simulink model "scarsModel"  (R2019b)
settings: Solver=ode14x  StartTime=0.0  StopTime=2000  FixedStep=0.1  MaxStep=1  MinStep=dT  RelTol=1e-3
model workspace (MAT data in the model file):
  actuators = 0
undefined symbols (not defined in the file): decsec, decstart, forcesBody, gyro, initMoments, L_mt, mag_sat, momentsBody, mt_gain, R_mt, refEuler, refVel, sun_position, TFinal, thruster, WMM2000
libraries: scars_library x15, simulink x3, vrlib x3, simulink_extras x2, aerolibnav x2, aerolibgravity2 x2, sharedtransform x2, aerolibutil x2, sharedutil x2
settings Model: OrderedModelArguments=off  Creator=asmialek  LastModifiedBy=asmialek
settings DataIOCC: SaveFormat=Array  ReturnWorkspaceOutputsName=scars_out

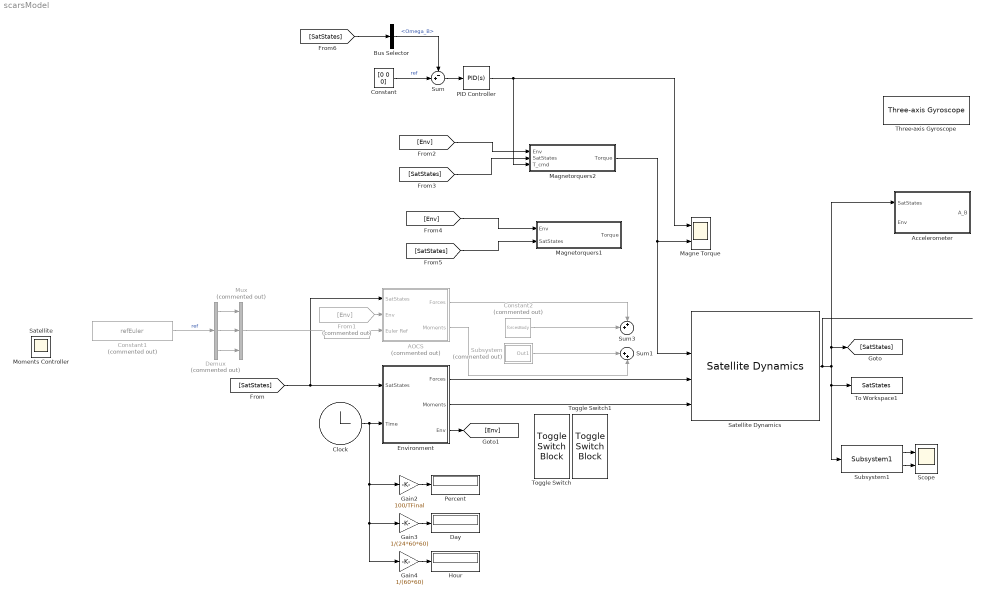
== system scarsModel ==
  AOCS : Subsystem  Commented=on
  Accelerometer : Subsystem
  Bus Selector : BusSelector  OutputSignals=Omega_B
  Clock : Clock
  Constant : Constant  Value=[0 0 0]
  Constant1 : Constant  Commented=on  Value=refEuler
  Constant2 : Constant  Commented=on  Value=forcesBody
  Day : Display
  Demux : Demux  Commented=on  Outputs=3
  "Environment " : Subsystem
  From1 : From  Commented=on  GotoTag=Env
  Gain2 : Gain  Gain=100/TFinal
  Gain3 : Gain  Gain=1/(24*60*60)
  Gain4 : Gain  Gain=1/(60*60)
  Hour : Display
  Magne Torque : Scope  NumInputPorts=2
  Magnetorquers1 : Subsystem
  Magnetorquers2 : Subsystem
  Mux : Mux  Commented=on  Inputs=3
  PID Controller : simulink/Continuous/PID Controller  Controller=PID  Form=Parallel  TimeDomain=Continuous-time  SampleTime=-1  IntegratorMethod=Forward Euler  FilterMethod=Forward Euler  ControllerParametersSource=internal  P=0.01  I=0  D=0.1  UseFilter=on  N=100  TunerSelectOption=Transfer Function Based (PID Tuner App)  InitialConditionSource=internal  InitialConditionForIntegrator=0  InitialConditionForFilter=0  DifferentiatorICPrevScaledInput=0  ExternalReset=none  TrackingMode=off  Kt=1  LimitOutput=off  UpperSaturationLimit=inf  LowerSaturationLimit=-inf  LinearizeAsGain=on  AntiWindupMode=none  Kb=1  POutMin=[]  POutMax=[]  IOutMin=[]  IOutMax=[]  DOutMin=[]  DOutMax=[]  NOutMin=[]  NOutMax=[]  SumOutMin=[]  SumOutMax=[]  SaturationOutMin=[]  SaturationOutMax=[]  PParamMin=[]  PParamMax=[]  IParamMin=[]  IParamMax=[]  DParamMin=[]  DParamMax=[]  NParamMin=[]  NParamMax=[]  KbParamMin=[]  KbParamMax=[]  KtParamMin=[]  KtParamMax=[]  KbOutMin=[]  KbOutMax=[]  KtOutMin=[]  KtOutMax=[]  IntegratorOutMin=[]  IntegratorOutMax=[]  FilterOutMin=[]  FilterOutMax=[]  SumI1OutMin=[]  SumI1OutMax=[]  SumI2OutMin=[]  SumI2OutMax=[]  SumI3OutMin=[]  SumI3OutMax=[]  SumI4OutMin=[]  SumI4OutMax=[]  SumDOutMin=[]  SumDOutMax=[]  DifferentiatorOutMin=[]  DifferentiatorOutMax=[]  FilterDiffOutCoefMin=[]  FilterDiffOutCoefMax=[]  ReciprocalOutMin=[]  ReciprocalOutMax=[]  SumDenOutMin=[]  SumDenOutMax=[]  SumNumOutMin=[]  SumNumOutMax=[]  DivideOutMin=[]  DivideOutMax=[]  IntegratorContinuousStateAttributes=''  IntegratorStateMustResolveToSignalObject=off  IntegratorRTWStateStorageClass=Auto  FilterContinuousStateAttributes=''  FilterStateMustResolveToSignalObject=off  FilterRTWStateStorageClass=Auto  ParallelPVariant=InternalParameters  IdealPVariant=Disabled  IVariant=InternalParameters  DVariant=InternalParameters  IntegratorVariant=Continuous  SatVariant=Disabled  AWVariant=Passthrough  PCopyVariant=Disabled  TRVariant=Disabled  FdbkBlocksVariant=Forward  IdealPFdbkVariant=Disabled  SatFdbkVariant=Disabled  DerivativeFilterVariant=ContFilter  NVariant=InternalParameters  NCopyVariant=Disabled  FilterICVariant=InternalICsFilter  IntegratorICVariant=InternalICs  ExternalResetVariant=Disabled  TRSumVariant=Passthrough  SumFdbkVariant=Disabled  SumVariant=Sum_PID
  Percent : Display
  Satellite Dynamics : scars_library/Advanced/Satellite Dynamics  Parameter4=Keplerian Elements  epoch=0  mass=0  a=6356e3+400e3  e=0  incl=0  RA=0  w=0  TA=0  initEuler=[0 0 0]  initEulerRates=[0 0 0]  TA_copy=0  TA_copy_copy=0  TA_copy_copy_copy=[10 25]  TA_copy_copy_copy_copy=[10 25]  initEuler_copy=[0 0 0]  initEulerRates_copy=[0 0 0]
      link override Moments Switch/Moments: Value=1
  Scope : Scope  NumInputPorts=2
  Subsystem : Subsystem  Commented=on
  Subsystem1 : scars_library/Subsystem1  SystemSampleTime=-1  Latency=0  AutoFrameSizeCalculation=off
  Sum : Sum  Inputs=-+|
  Sum1 : Sum  Inputs=|++
  Sum3 : Sum  Inputs=++|
  Three-axis Gyroscope : aerolibnav/Three-axis Gyroscope  dtype_g=on  w_g=190  z_g=0.707  g_sf_cc=[1 0 0; 0 1 0; 0 0 1]  g_bias=[0 0 0]  g_sen=[0 0 0]  g_Ts=0  g_rand=on  g_seeds=[23093 23094 23095]  g_pow=[0.0001 0.0001 0.0001]  g_sat="[-inf  -inf  -inf  inf inf inf]"
      settings: SourceProductName=Aerospace Blockset  SourceProductBaseCode=AE
  To Workspace1 : ToWorkspace  VariableName=SatStates  SaveFormat=Timeseries  SampleTime=-1
  Toggle Switch : ToggleSwitchBlock
      settings: Values={{'Off', 'On'}, [0 1]}
  Toggle Switch1 : ToggleSwitchBlock
      settings: Values={{'Off', 'On'}, [0 1]}
  Moments Controller : Scope
  Satellite : Scope
  wires:
  Constant2/1 -> Sum3/2
  [SatStates] -> AOCS/1(SatStates), "Environment "/1(SatStates)
  "Environment "/1(Forces) -> Satellite Dynamics/3
  "Environment "/2(Moments) -> Satellite Dynamics/4
  Subsystem/1(Out1) -> Sum1/1
  Clock/1 -> Gain4/1, Gain3/1, Gain2/1, "Environment "/2(Time)
  "Environment "/3(Env) -> [Env]
  From1/1 -> AOCS/2(Env)
  AOCS/1(Forces) -> Sum3/1
  AOCS/2(Moments) -> Sum1/2
  Gain2/1 -> Percent/1
  Gain3/1 -> Day/1
  Gain4/1 -> Hour/1
  Constant1/1 -> Demux/1  "ref"
  Demux/2 -> Mux/2
  Demux/3 -> Mux/3
  Demux/1 -> Mux/1
  Mux/1 -> AOCS/3(Euler Ref)
  [Env] -> Magnetorquers1/1(Env)
  [SatStates] -> Magnetorquers1/2(SatStates)
  [SatStates] -> Magnetorquers2/2(SatStates)
  [Env] -> Magnetorquers2/1(Env)
  Constant/1 -> Sum/2  "ref"
  Sum/1 -> PID Controller/1
  Bus Selector/1 -> Sum/1  "<Omega_B>"
  [SatStates] -> Bus Selector/1
  Magnetorquers2/1(Torque) -> Satellite Dynamics/2, Magne Torque/2
  PID Controller/1 -> Magne Torque/1, Magnetorquers2/3(T_cmd)
  Subsystem1/2 -> Scope/2
  Subsystem1/1 -> Scope/1
  Satellite Dynamics/1 -> Subsystem1/1, To Workspace1/1, Accelerometer/1(SatStates), [SatStates]

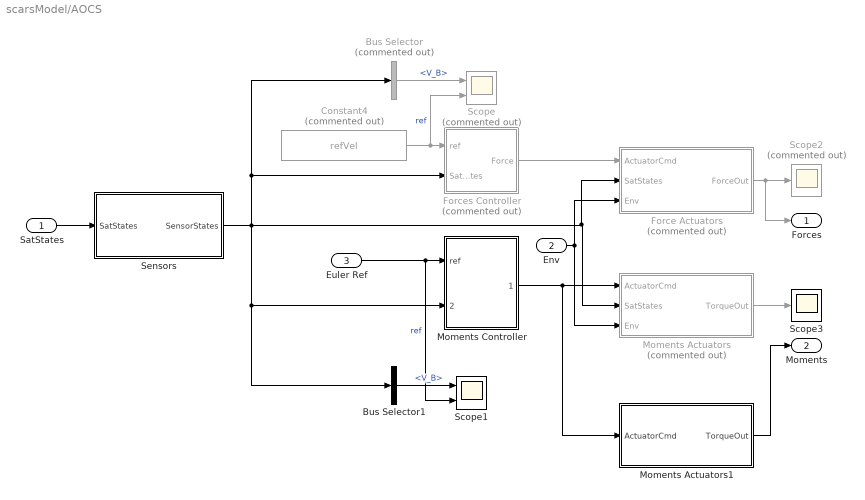
== system scarsModel/AOCS ==
  SatStates : Inport
  Env : Inport  Port=2
  Euler Ref : Inport  Port=3
  Bus Selector : BusSelector  Commented=on  OutputSignals=V_B
  Bus Selector1 : BusSelector  OutputSignals=V_B
  Constant4 : Constant  Commented=on  Value=refVel
  Force Actuators : Subsystem  Commented=on
  Forces Controller : Subsystem  Commented=on
  Moments Actuators : Subsystem  Commented=on
  Moments Actuators1 : Subsystem
  Moments Controller : Subsystem
  Scope : Scope  Commented=on  NumInputPorts=2
  Scope1 : Scope  NumInputPorts=2
  Scope2 : Scope  Commented=on
  Scope3 : Scope
  Sensors : Subsystem
  Forces : Outport
  Moments : Outport  Port=2
  wires:
  Force Actuators/1(ForceOut) -> Forces/1, Scope2/1
  SatStates/1 -> Sensors/1(SatStates)
  Constant4/1 -> Scope/2, Forces Controller/1(ref)  "ref"
  Forces Controller/1(Force) -> Force Actuators/1(ActuatorCmd)
  Euler Ref/1 -> Scope1/2, Moments Controller/1(ref)  "ref"
  Bus Selector/1 -> Scope/1  "<V_B>"
  Bus Selector1/1 -> Scope1/1  "<V_B>"
  Moments Actuators/1(TorqueOut) -> Scope3/1
  Sensors/1(SensorStates) -> Bus Selector/1, Forces Controller/2(SatStates), Force Actuators/2(SatStates), Moments Actuators/2(SatStates), Bus Selector1/1, Moments Controller/2(SatStates)
  Env/1 -> Force Actuators/3(Env), Moments Actuators/3(Env)
  Moments Controller/1(Torque) -> Moments Actuators1/1(ActuatorCmd), Moments Actuators/1(ActuatorCmd)
  Moments Actuators1/1(TorqueOut) -> Moments/1

== system scarsModel/Accelerometer ==
  SatStates : Inport
  Bus Element In : Inport  Port=2  PortName=Env  Element=Gravitational Force [N]
  Bus Selector : BusSelector  OutputSignals=A_B,Omega_B,dOmega_B/dt
  Constant : Constant  Value=[0 0 0]
  Three-axis Accelerometer : aerolibnav/Three-axis Accelerometer  units=Metric (MKS)  acc=[0 0 0]  gtype=on  dtype_a=on  w_a=190  z_a=0.707  a_sf_cc=[1 0 0; 0 1 0; 0 0 1]  a_bias=[0 0 0]  a_Ts=0  a_rand=on  a_seeds=[23093 23094 23095]  a_pow=[0.001 0.001 0.001]  a_sat="[-inf  -inf  -inf  inf inf inf]"
      settings: SourceProductName=Aerospace Blockset  SourceProductBaseCode=AE
  A_B : Outport
  wires:
  SatStates/1 -> Bus Selector/1
  Constant/1 -> Three-axis Accelerometer/4
  Bus Selector/1 -> Three-axis Accelerometer/1  "<A_B>"
  Bus Selector/2 -> Three-axis Accelerometer/2  "<Omega_B>"
  Bus Selector/3 -> Three-axis Accelerometer/3  "<dOmega_B/dt>"
  Bus Element In/1 -> Three-axis Accelerometer/5
  Three-axis Accelerometer/1 -> A_B/1

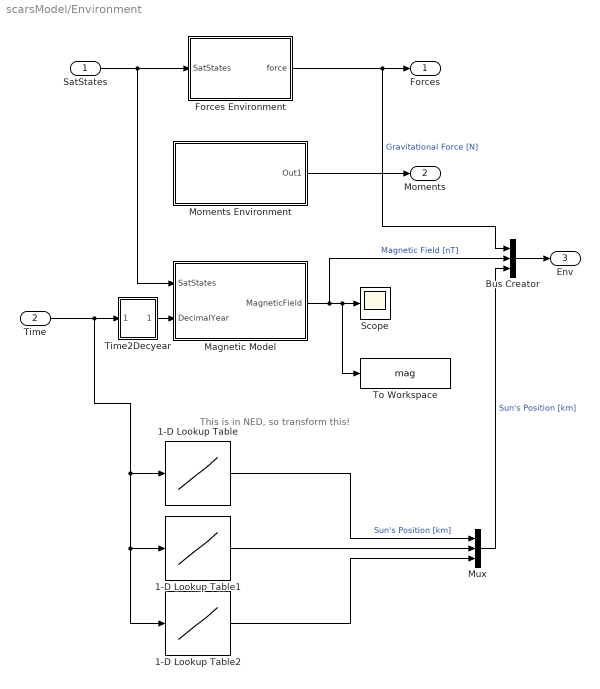
== system scarsModel/Environment  ==
  note: This is in NED, so transform this!
  SatStates : Inport
  Time : Inport  Port=2
  1-D Lookup Table : Lookup_n-D  NumberOfTableDimensions=1  BreakpointsForDimension1=sun_position(:,1)  Table=sun_position(:,2)  InternalRulePriority=Speed  RndMeth=Simplest  InputSameDT=on
  1-D Lookup Table1 : Lookup_n-D  NumberOfTableDimensions=1  BreakpointsForDimension1=sun_position(:,1)  Table=sun_position(:,3)  InternalRulePriority=Speed  RndMeth=Simplest  InputSameDT=on
  1-D Lookup Table2 : Lookup_n-D  NumberOfTableDimensions=1  BreakpointsForDimension1=sun_position(:,1)  Table=sun_position(:,4)  InternalRulePriority=Speed  RndMeth=Simplest  InputSameDT=on
  Bus Creator : BusCreator  Inputs=3
  Forces Environment : Subsystem
  Magnetic Model : Subsystem
  Moments Environment : Subsystem
  Mux : Mux  Inputs=3
  Scope : Scope
  Time2Decyear : Subsystem
  To Workspace : ToWorkspace  VariableName=mag  SampleTime=-1
  Forces : Outport
  Moments : Outport  Port=2
  Env : Outport  Port=3
  wires:
  SatStates/1 -> Forces Environment/1(SatStates), Magnetic Model/1(SatStates)
  Forces Environment/1(force) -> Bus Creator/1, Forces/1  "Gravitational Force [N]"
  Moments Environment/1(Out1) -> Moments/1
  Time2Decyear/1("  ") -> Magnetic Model/2(DecimalYear)
  Magnetic Model/1(MagneticField) -> Bus Creator/2, To Workspace/1, Scope/1  "Magnetic Field [nT]"
  Bus Creator/1 -> Env/1
  1-D Lookup Table2/1 -> Mux/3
  Time/1 -> 1-D Lookup Table2/1, 1-D Lookup Table1/1, 1-D Lookup Table/1, Time2Decyear/1(" ")
  1-D Lookup Table/1 -> Mux/1  "Sun's Position [km]"
  1-D Lookup Table1/1 -> Mux/2
  Mux/1 -> Bus Creator/3  "Sun's Position [km]"

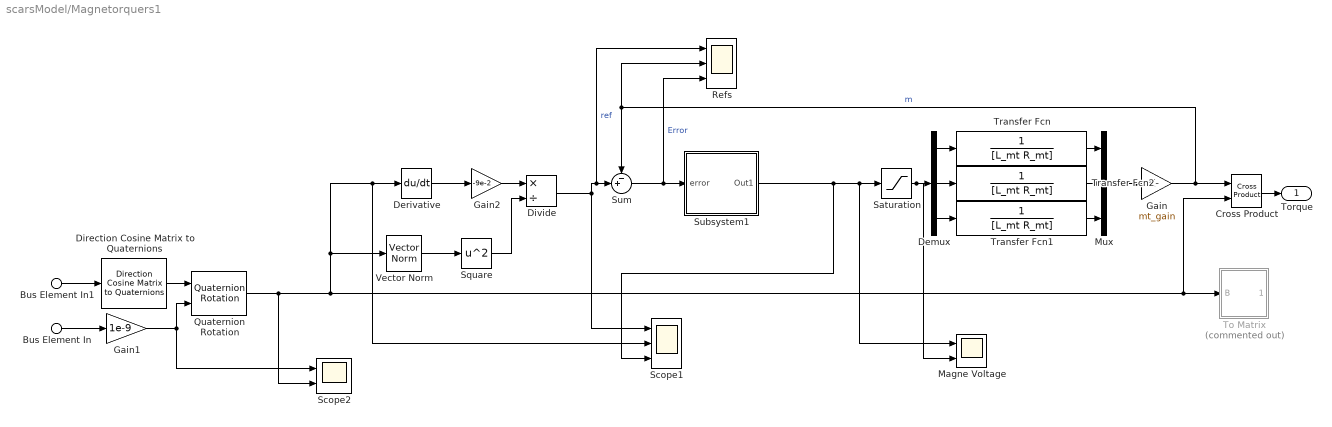
== system scarsModel/Magnetorquers1 ==
  Bus Element In : Inport  PortName=Env  Element=Magnetic Field [nT]
  Bus Element In1 : Inport  Port=2  PortName=SatStates  Element=DCM_NED2B
  Cross Product : vrlib/Utilities/Cross Product
      settings: SourceProductName=Simulink
  Demux : Demux  Outputs=3
  Derivative : Derivative
  Direction Cosine Matrix to Quaternions : sharedtransform/Direction Cosine Matrix  to Quaternions  aMode=0  action=None  tolerance=eps(2)
      settings: SourceProductName=Aerospace Blockset  SourceProductBaseCode=AE
  Divide : Product  Inputs=*/
  Gain : Gain  Gain=mt_gain
  Gain1 : Gain  Gain=1e-9
  Gain2 : Gain  Gain=-9e-2
  Magne Voltage : Scope  NumInputPorts=2
  Mux : Mux  Inputs=3
  Quaternion Rotation : aerolibutil/Quaternion Rotation
  Refs : Scope  NumInputPorts=3
  Saturation : Saturate  UpperLimit=mag_sat  LowerLimit=-mag_sat
  Scope1 : Scope  NumInputPorts=3
  Scope2 : Scope  NumInputPorts=2
  Square : Math  Operator=square  SignedPower=off  SaturateOnIntegerOverflow=on
  Subsystem1 : Subsystem
  Sum : Sum  Inputs=-+|
  To Matrix : Subsystem  Commented=on
  Transfer Fcn : TransferFcn  Denominator=[L_mt R_mt]
  Transfer Fcn1 : TransferFcn  Denominator=[L_mt R_mt]
  Transfer Fcn2 : TransferFcn  Denominator=[L_mt R_mt]
  Vector Norm : scars_library/Vector Norm  SystemSampleTime=-1  Latency=0  AutoFrameSizeCalculation=off
  Torque : Outport
  wires:
  Gain1/1 -> Quaternion Rotation/2, Scope2/1
  Saturation/1 -> Magne Voltage/2, Demux/1
  Gain/1 -> Cross Product/1, Refs/2, Sum/1  "m"
  Cross Product/1 -> Torque/1
  Direction Cosine Matrix to Quaternions/1 -> Quaternion Rotation/1
  Bus Element In1/1 -> Direction Cosine Matrix to Quaternions/1
  Bus Element In/1 -> Gain1/1
  Demux/3 -> Transfer Fcn1/1
  Demux/2 -> Transfer Fcn2/1
  Demux/1 -> Transfer Fcn/1
  Transfer Fcn2/1 -> Mux/2
  Transfer Fcn1/1 -> Mux/3
  Transfer Fcn/1 -> Mux/1
  Mux/1 -> Gain/1
  Vector Norm/1 -> Square/1
  Square/1 -> Divide/2
  Quaternion Rotation/1 -> Scope1/2, Derivative/1, Vector Norm/1, To Matrix/1(B), Cross Product/2, Scope2/2
  Derivative/1 -> Gain2/1
  Sum/1 -> Refs/3, Subsystem1/1(error)  "Error"
  Gain2/1 -> Divide/1
  Subsystem1/1(Out1) -> Magne Voltage/1, Saturation/1, Scope1/3
  Divide/1 -> Scope1/1, Refs/1, Sum/2  "ref"

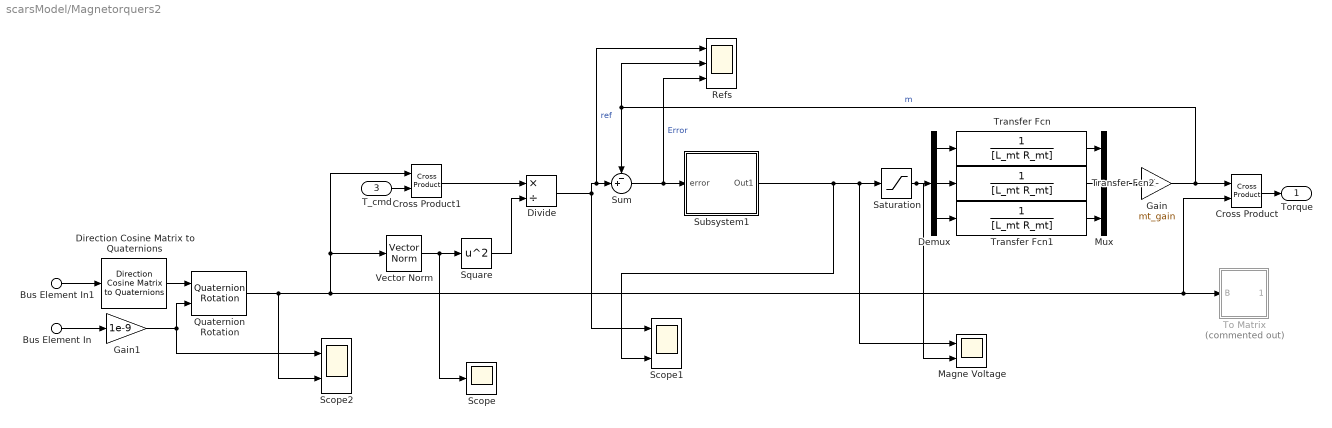
== system scarsModel/Magnetorquers2 ==
  Bus Element In : Inport  PortName=Env  Element=Magnetic Field [nT]
  Bus Element In1 : Inport  Port=2  PortName=SatStates  Element=DCM_NED2B
  T_cmd : Inport  Port=3
  Cross Product : vrlib/Utilities/Cross Product
      settings: SourceProductName=Simulink
  Cross Product1 : vrlib/Utilities/Cross Product
      settings: SourceProductName=Simulink
  Demux : Demux  Outputs=3
  Direction Cosine Matrix to Quaternions : sharedtransform/Direction Cosine Matrix  to Quaternions  aMode=0  action=None  tolerance=eps(2)
      settings: SourceProductName=Aerospace Blockset  SourceProductBaseCode=AE
  Divide : Product  Inputs=*/
  Gain : Gain  Gain=mt_gain
  Gain1 : Gain  Gain=1e-9
  Magne Voltage : Scope  NumInputPorts=2
  Mux : Mux  Inputs=3
  Quaternion Rotation : aerolibutil/Quaternion Rotation
  Refs : Scope  NumInputPorts=3
  Saturation : Saturate  UpperLimit=mag_sat  LowerLimit=-mag_sat
  Scope : Scope
  Scope1 : Scope  NumInputPorts=3
  Scope2 : Scope  NumInputPorts=2
  Square : Math  Operator=square  SignedPower=off  SaturateOnIntegerOverflow=on
  Subsystem1 : Subsystem
  Sum : Sum  Inputs=-+|
  To Matrix : Subsystem  Commented=on
  Transfer Fcn : TransferFcn  Denominator=[L_mt R_mt]
  Transfer Fcn1 : TransferFcn  Denominator=[L_mt R_mt]
  Transfer Fcn2 : TransferFcn  Denominator=[L_mt R_mt]
  Vector Norm : scars_library/Vector Norm  SystemSampleTime=-1  Latency=0  AutoFrameSizeCalculation=off
  Torque : Outport
  wires:
  Divide/1 -> Sum/2, Refs/1, Scope1/1  "ref"
  Subsystem1/1(Out1) -> Scope1/3, Saturation/1, Magne Voltage/1
  Cross Product1/1 -> Divide/1
  Sum/1 -> Subsystem1/1(error), Refs/3  "Error"
  Quaternion Rotation/1 -> Scope2/2, Cross Product/2, To Matrix/1(B), Cross Product1/1, Vector Norm/1
  Square/1 -> Divide/2
  Vector Norm/1 -> Scope/1, Square/1
  Mux/1 -> Gain/1
  Transfer Fcn/1 -> Mux/1
  Transfer Fcn1/1 -> Mux/3
  Transfer Fcn2/1 -> Mux/2
  Demux/1 -> Transfer Fcn/1
  Demux/2 -> Transfer Fcn2/1
  Demux/3 -> Transfer Fcn1/1
  Bus Element In/1 -> Gain1/1
  Bus Element In1/1 -> Direction Cosine Matrix to Quaternions/1
  Direction Cosine Matrix to Quaternions/1 -> Quaternion Rotation/1
  Cross Product/1 -> Torque/1
  Gain/1 -> Sum/1, Refs/2, Cross Product/1  "m"
  Saturation/1 -> Demux/1, Magne Voltage/2
  Gain1/1 -> Scope2/1, Quaternion Rotation/2
  T_cmd/1 -> Cross Product1/2

== system scarsModel/Subsystem ==
  Constant1 : Constant  Value=momentsBody
  Constant2 : Constant  Value=momentsBody
  Gain : Gain  Gain=-1
  Sum : Sum  Inputs=|++
  Out1 : Outport
  wires:
  Constant1/1 -> Sum/1
  Sum/1 -> Out1/1
  Gain/1 -> Sum/2
  Constant2/1 -> Gain/1

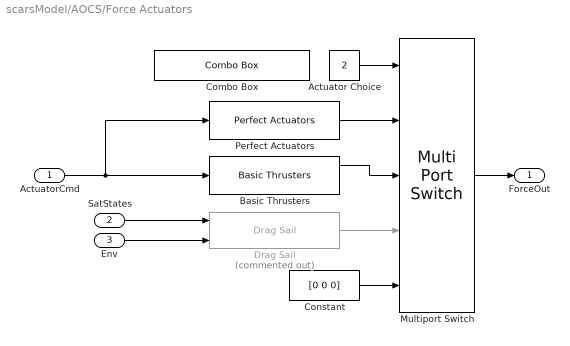
== system scarsModel/AOCS/Force Actuators ==
  ActuatorCmd : Inport
  SatStates : Inport  Port=2
  Env : Inport  Port=3
  Actuator Choice : Constant  Value=2
  Basic Thrusters : scars_library/Actuators/Basic Thrusters  delay=0  thrust_max=0  thrust_min=0  power=0
  Combo Box : ComboBox  LabelPosition=Hide  SelectedLabel=Thrusters
      settings: Values={{'Perfect Actuators', 'Thrusters', 'idontknowyet', 'No Actuators'}, [1 2 3 4]}
  Constant : Constant  Value=[0 0 0]
  Drag Sail : scars_library/Actuators/Drag Sail  Commented=on  SystemSampleTime=-1  Latency=0  AutoFrameSizeCalculation=off
  Multiport Switch : MultiPortSwitch  Inputs=4  DiagnosticForDefault=Warning
  Perfect Actuators : scars_library/Actuators/Perfect Actuators  k=1
  ForceOut : Outport
  wires:
  Perfect Actuators/1 -> Multiport Switch/2
  Constant/1 -> Multiport Switch/5
  Actuator Choice/1 -> Multiport Switch/1
  ActuatorCmd/1 -> Perfect Actuators/1, Basic Thrusters/1
  Multiport Switch/1 -> ForceOut/1
  Drag Sail/1 -> Multiport Switch/4
  Basic Thrusters/1 -> Multiport Switch/3
  Env/1 -> Drag Sail/2
  SatStates/1 -> Drag Sail/1

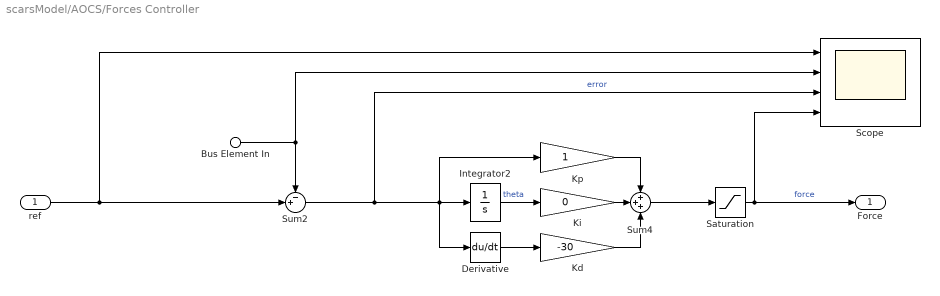
== system scarsModel/AOCS/Forces Controller ==
  ref : Inport
  Bus Element In : Inport  Port=2  PortName=SatStates  Element=V_B
  Derivative : Derivative
  Integrator2 : Integrator
  Kd : Gain  Gain=-30
  Ki : Gain  Gain=0
  Kp : Gain
  Saturation : Saturate  UpperLimit=3  LowerLimit=-3
  Scope : Scope  NumInputPorts=4
  Sum2 : Sum  Inputs=-+|
  Sum4 : Sum  Inputs=+++
  Force : Outport
  wires:
  Saturation/1 -> Force/1, Scope/4  "force"
  ref/1 -> Sum2/2, Scope/1
  Sum4/1 -> Saturation/1
  Bus Element In/1 -> Sum2/1, Scope/2
  Kd/1 -> Sum4/3
  Kp/1 -> Sum4/1
  Sum2/1 -> Kp/1, Derivative/1, Integrator2/1, Scope/3  "error"
  Ki/1 -> Sum4/2
  Derivative/1 -> Kd/1
  Integrator2/1 -> Ki/1  "theta"

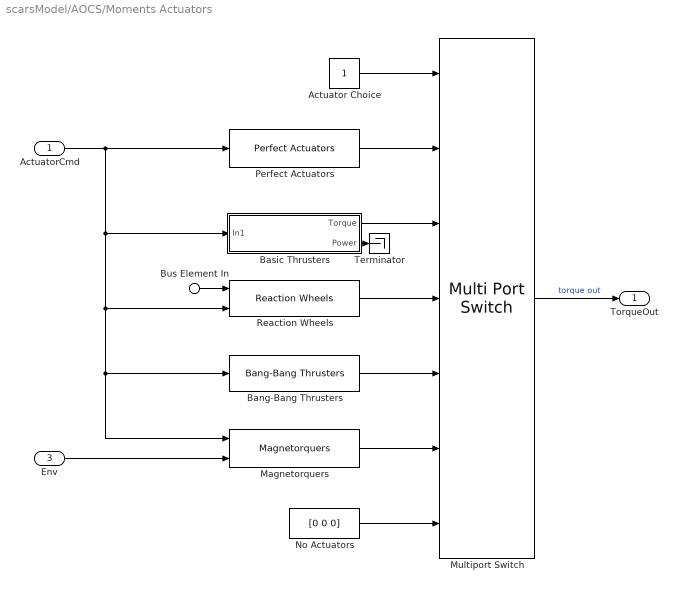
== system scarsModel/AOCS/Moments Actuators ==
  ActuatorCmd : Inport
  Bus Element In : Inport  Port=2  PortName=SatStates  Element=V_B
  Env : Inport  Port=3
  Actuator Choice : Constant
  Bang-Bang Thrusters : scars_library/Actuators/Bang-Bang Thrusters  SystemSampleTime=-1  Latency=0  AutoFrameSizeCalculation=off
  Basic Thrusters : Subsystem
  Magnetorquers : scars_library/Actuators/Magnetorquers  SystemSampleTime=-1  Latency=0  AutoFrameSizeCalculation=off
  Multiport Switch : MultiPortSwitch  Inputs=6  DiagnosticForDefault=Warning
  No Actuators : Constant  Value=[0 0 0]
  Perfect Actuators : scars_library/Actuators/Perfect Actuators  SystemSampleTime=-1  Latency=0  AutoFrameSizeCalculation=off
  Reaction Wheels : scars_library/Actuators/Reaction Wheels  SystemSampleTime=-1  Latency=0  AutoFrameSizeCalculation=off
  Terminator : Terminator
  TorqueOut : Outport
  wires:
  Perfect Actuators/1 -> Multiport Switch/2
  Bang-Bang Thrusters/1 -> Multiport Switch/5
  Actuator Choice/1 -> Multiport Switch/1
  Reaction Wheels/1 -> Multiport Switch/4
  Multiport Switch/1 -> TorqueOut/1  "torque out"
  ActuatorCmd/1 -> Perfect Actuators/1, Basic Thrusters/1(In1), Reaction Wheels/2, Magnetorquers/1, Bang-Bang Thrusters/1
  Bus Element In/1 -> Reaction Wheels/1
  Basic Thrusters/1(Torque) -> Multiport Switch/3
  No Actuators/1 -> Multiport Switch/7
  Magnetorquers/1 -> Multiport Switch/6
  Basic Thrusters/2(Power) -> Terminator/1
  Env/1 -> Magnetorquers/2

== system scarsModel/AOCS/Moments Actuators1 ==
  ActuatorCmd : Inport
  Perfect Actuators : scars_library/Actuators/Perfect Actuators  k=1
  TorqueOut : Outport
  wires:
  ActuatorCmd/1 -> Perfect Actuators/1
  Perfect Actuators/1 -> TorqueOut/1

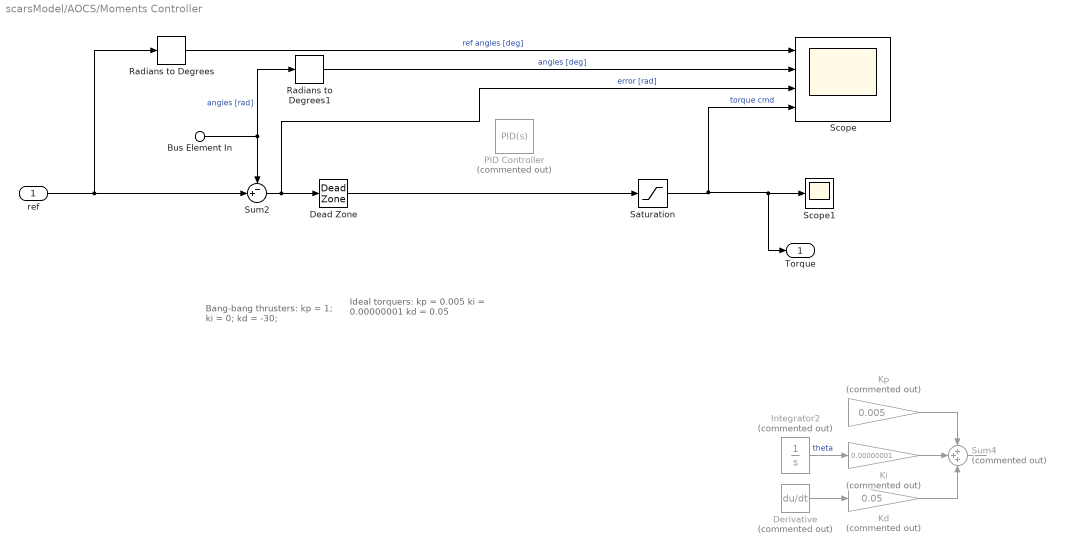
== system scarsModel/AOCS/Moments Controller ==
  note: Ideal torquers:
      | kp = 0.005
      | ki = 0.00000001
      | kd = 0.05
  note: Bang-bang thrusters:
      | kp = 1;
      | ki = 0;
      | kd = -30;
  ref : Inport
  Bus Element In : Inport  Port=2  PortName=SatStates  Element=V_B
  Dead Zone : DeadZone  LowerValue=-1e-3  UpperValue=1e-3  SaturateOnIntegerOverflow=on
  Derivative : Derivative  Commented=on
  Integrator2 : Integrator  Commented=on
  Kd : Gain  Commented=on  Gain=0.05
  Ki : Gain  Commented=on  Gain=0.00000001
  Kp : Gain  Commented=on  Gain=0.005
  PID Controller : simulink/Continuous/PID Controller  Commented=on  Controller=PID  Form=Parallel  TimeDomain=Continuous-time  SampleTime=-1  IntegratorMethod=Forward Euler  FilterMethod=Forward Euler  ControllerParametersSource=internal  P=0.005  I=0.00000001  D=0.05  UseFilter=on  N=100  TunerSelectOption=Transfer Function Based (PID Tuner App)  InitialConditionSource=internal  InitialConditionForIntegrator=0  InitialConditionForFilter=0  DifferentiatorICPrevScaledInput=0  ExternalReset=none  TrackingMode=off  Kt=1  LimitOutput=off  UpperSaturationLimit=inf  LowerSaturationLimit=-inf  LinearizeAsGain=on  AntiWindupMode=none  Kb=1  POutMin=[]  POutMax=[]  IOutMin=[]  IOutMax=[]  DOutMin=[]  DOutMax=[]  NOutMin=[]  NOutMax=[]  SumOutMin=[]  SumOutMax=[]  SaturationOutMin=[]  SaturationOutMax=[]  PParamMin=[]  PParamMax=[]  IParamMin=[]  IParamMax=[]  DParamMin=[]  DParamMax=[]  NParamMin=[]  NParamMax=[]  KbParamMin=[]  KbParamMax=[]  KtParamMin=[]  KtParamMax=[]  KbOutMin=[]  KbOutMax=[]  KtOutMin=[]  KtOutMax=[]  IntegratorOutMin=[]  IntegratorOutMax=[]  FilterOutMin=[]  FilterOutMax=[]  SumI1OutMin=[]  SumI1OutMax=[]  SumI2OutMin=[]  SumI2OutMax=[]  SumI3OutMin=[]  SumI3OutMax=[]  SumI4OutMin=[]  SumI4OutMax=[]  SumDOutMin=[]  SumDOutMax=[]  DifferentiatorOutMin=[]  DifferentiatorOutMax=[]  FilterDiffOutCoefMin=[]  FilterDiffOutCoefMax=[]  ReciprocalOutMin=[]  ReciprocalOutMax=[]  SumDenOutMin=[]  SumDenOutMax=[]  SumNumOutMin=[]  SumNumOutMax=[]  DivideOutMin=[]  DivideOutMax=[]  IntegratorContinuousStateAttributes=''  IntegratorStateMustResolveToSignalObject=off  IntegratorRTWStateStorageClass=Auto  FilterContinuousStateAttributes=''  FilterStateMustResolveToSignalObject=off  FilterRTWStateStorageClass=Auto  ParallelPVariant=InternalParameters  IdealPVariant=Disabled  IVariant=InternalParameters  DVariant=InternalParameters  IntegratorVariant=Continuous  SatVariant=Disabled  AWVariant=Passthrough  PCopyVariant=Disabled  TRVariant=Disabled  FdbkBlocksVariant=Forward  IdealPFdbkVariant=Disabled  SatFdbkVariant=Disabled  DerivativeFilterVariant=ContFilter  NVariant=InternalParameters  NCopyVariant=Disabled  FilterICVariant=InternalICsFilter  IntegratorICVariant=InternalICs  ExternalResetVariant=Disabled  TRSumVariant=Passthrough  SumFdbkVariant=Disabled  SumVariant=Sum_PID
  Radians to Degrees : simulink_extras/Transformations/Radians to Degrees
  Radians to Degrees1 : simulink_extras/Transformations/Radians to Degrees
  Saturation : Saturate  UpperLimit=3  LowerLimit=-3
  Scope : Scope  NumInputPorts=4
  Scope1 : Scope
  Sum2 : Sum  Inputs=-+|
  Sum4 : Sum  Commented=on  Inputs=+++
  Torque : Outport
  wires:
  Saturation/1 -> Torque/1, Scope1/1, Scope/4  "torque cmd"
  ref/1 -> Sum2/2, Radians to Degrees/1
  Bus Element In/1 -> Sum2/1, Radians to Degrees1/1  "angles [rad]"
  Radians to Degrees/1 -> Scope/1  "ref angles [deg]"
  Radians to Degrees1/1 -> Scope/2  "angles [deg]"
  Sum2/1 -> Scope/3, Dead Zone/1  "error [rad]"
  Ki/1 -> Sum4/2
  ? -> Kp/1, Derivative/1, Integrator2/1
  Sum4/1 -> ?
  Kp/1 -> Sum4/1
  Kd/1 -> Sum4/3
  Integrator2/1 -> Ki/1  "theta"
  Derivative/1 -> Kd/1
  Dead Zone/1 -> Saturation/1

== system scarsModel/AOCS/Sensors ==
  SatStates : Inport
  Bus Creator : BusCreator  Inputs=9
  Bus Selector : BusSelector  OutputSignals=V_ecef,X_ecef,V_B,Euler_NED,Omega_B,lla,ECI2Body,ECEF2NED,NED2Body
  Gyros : Subsystem  Commented=through
  SensorStates : Outport
  wires:
  SatStates/1 -> Bus Selector/1
  Bus Creator/1 -> SensorStates/1
  Bus Selector/7 -> Bus Creator/7  "<ECI2Body>"
  Bus Selector/8 -> Bus Creator/8  "<ECEF2NED>"
  Bus Selector/9 -> Bus Creator/9  "<NED2Body>"
  Bus Selector/6 -> Bus Creator/6  "<lla>"
  Bus Selector/5 -> Gyros/1(In1)  "<Omega_B>"
  Bus Selector/1 -> Bus Creator/1  "<V_ecef>"
  Gyros/1(Out1) -> Bus Creator/5  "Omega_body"
  Bus Selector/2 -> Bus Creator/2  "<X_ecef>"
  Bus Selector/3 -> Bus Creator/3  "<V_B>"
  Bus Selector/4 -> Bus Creator/4  "<Euler_NED>"

== system scarsModel/Environment /Forces Environment ==
  SatStates : Inport
  Subsystem : Subsystem
  force : Outport
  wires:
  Subsystem/1(Out1) -> force/1
  SatStates/1 -> Subsystem/1(SatStates)

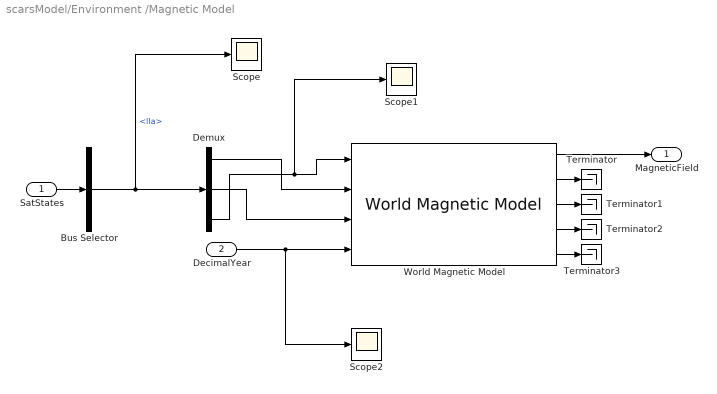
== system scarsModel/Environment /Magnetic Model ==
  SatStates : Inport
  DecimalYear : Inport  Port=2
  Bus Selector : BusSelector  OutputSignals=lla
  Demux : Demux  Outputs=3
  Scope : Scope
  Scope1 : Scope
  Scope2 : Scope
  Terminator{,1..3} (4 alike) : Terminator
  World Magnetic Model : aerolibgravity2/World Magnetic Model  model=WMM2000 (2000-2005)  customFile='WMM2015v2.COF'  units=Metric (MKS)  time_in=on  month=January  day=1  year=2015  action=Error  h_out=on  dec_out=on  inc_out=on  ti_out=on
      settings: SourceProductName=Aerospace Blockset  SourceProductBaseCode=AE
  MagneticField : Outport
  wires:
  SatStates/1 -> Bus Selector/1
  DecimalYear/1 -> Scope2/1, World Magnetic Model/4
  World Magnetic Model/1 -> MagneticField/1
  World Magnetic Model/2 -> Terminator/1
  World Magnetic Model/5 -> Terminator3/1
  World Magnetic Model/3 -> Terminator1/1
  World Magnetic Model/4 -> Terminator2/1
  Bus Selector/1 -> Demux/1, Scope/1  "<lla>"
  Demux/1 -> World Magnetic Model/2
  Demux/2 -> World Magnetic Model/3
  Demux/3 -> Scope1/1, World Magnetic Model/1

== system scarsModel/Environment /Moments Environment ==
  Constant : Constant  Value=initMoments
  Out1 : Outport
  wires:
  Constant/1 -> Out1/1

== system scarsModel/Environment /Time2Decyear ==
  " " : Inport
  Decsec : Gain  Gain=decsec
  Initial Decyear : Constant  Value=decstart
  Sum : Sum  Inputs=|++
  "  " : Outport
  wires:
  Initial Decyear/1 -> Sum/1
  " "/1 -> Decsec/1
  Decsec/1 -> Sum/2
  Sum/1 -> "  "/1

== system scarsModel/Magnetorquers1/Subsystem1 ==
  error : Inport
  Derivative : Derivative
  Integrator2 : Integrator
  Kd : Gain  Gain=0
  Ki : Gain  Gain=0.001
  Kp : Gain
  Magne PID : Scope  NumInputPorts=3
  Saturation : Saturate  UpperLimit=1  LowerLimit=-1
  Sum4 : Sum  Inputs=+++
  Out1 : Outport
  wires:
  error/1 -> Kp/1, Derivative/1, Integrator2/1
  Integrator2/1 -> Ki/1  "theta"
  Sum4/1 -> Out1/1
  Kp/1 -> Magne PID/1, Sum4/1
  Ki/1 -> Saturation/1
  Derivative/1 -> Kd/1
  Kd/1 -> Magne PID/3, Sum4/3
  Saturation/1 -> Magne PID/2, Sum4/2

== system scarsModel/Magnetorquers1/To Matrix ==
  B : Inport
  Constant : Constant  Value=0
  Constant1 : Constant  Value=0
  Constant2 : Constant  Value=0
  Create 3x3 Matrix : sharedutil/Create 3x3 Matrix  aMode=aMode
  Demux : Demux  Outputs=3
  Gain1 : Gain  Gain=-1
  Gain2 : Gain  Gain=-1
  Gain3 : Gain  Gain=-1
  B_3x3 : Outport
  wires:
  Constant1/1 -> Create 3x3 Matrix/5
  Gain1/1 -> Create 3x3 Matrix/3
  B/1 -> Demux/1
  Demux/1 -> Create 3x3 Matrix/6, Gain3/1
  Demux/2 -> Gain1/1, Create 3x3 Matrix/7
  Constant2/1 -> Create 3x3 Matrix/9
  Create 3x3 Matrix/1 -> B_3x3/1
  Gain3/1 -> Create 3x3 Matrix/8
  Gain2/1 -> Create 3x3 Matrix/4
  Demux/3 -> Gain2/1, Create 3x3 Matrix/2
  Constant/1 -> Create 3x3 Matrix/1

== system scarsModel/Magnetorquers2/Subsystem1 ==
  error : Inport
  Derivative : Derivative
  Integrator2 : Integrator
  Kd : Gain  Gain=0.001
  Ki : Gain  Gain=0.001
  Kp : Gain
  Magne PID : Scope  NumInputPorts=3
  Saturation : Saturate  UpperLimit=1  LowerLimit=-1
  Sum4 : Sum  Inputs=+++
  Out1 : Outport
  wires:
  Saturation/1 -> Sum4/2, Magne PID/2
  Kd/1 -> Sum4/3, Magne PID/3
  Derivative/1 -> Kd/1
  Ki/1 -> Saturation/1
  Kp/1 -> Sum4/1, Magne PID/1
  Sum4/1 -> Out1/1
  Integrator2/1 -> Ki/1  "theta"
  error/1 -> Integrator2/1, Derivative/1, Kp/1

== system scarsModel/Magnetorquers2/To Matrix ==
  B : Inport
  Constant : Constant  Value=0
  Constant1 : Constant  Value=0
  Constant2 : Constant  Value=0
  Create 3x3 Matrix : sharedutil/Create 3x3 Matrix  aMode=aMode
  Demux : Demux  Outputs=3
  Gain1 : Gain  Gain=-1
  Gain2 : Gain  Gain=-1
  Gain3 : Gain  Gain=-1
  B_3x3 : Outport
  wires:
  Constant/1 -> Create 3x3 Matrix/1
  Demux/3 -> Create 3x3 Matrix/2, Gain2/1
  Gain2/1 -> Create 3x3 Matrix/4
  Gain3/1 -> Create 3x3 Matrix/8
  Create 3x3 Matrix/1 -> B_3x3/1
  Constant2/1 -> Create 3x3 Matrix/9
  Demux/2 -> Create 3x3 Matrix/7, Gain1/1
  Demux/1 -> Gain3/1, Create 3x3 Matrix/6
  B/1 -> Demux/1
  Gain1/1 -> Create 3x3 Matrix/3
  Constant1/1 -> Create 3x3 Matrix/5

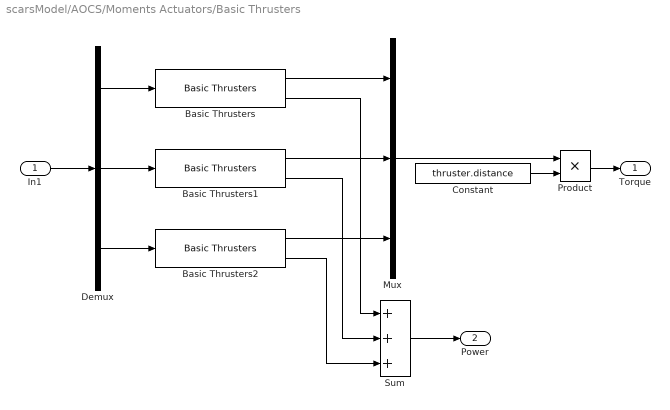
== system scarsModel/AOCS/Moments Actuators/Basic Thrusters ==
  In1 : Inport
  Basic Thrusters : scars_library/Actuators/Basic Thrusters  SystemSampleTime=-1  Latency=0  AutoFrameSizeCalculation=off
  Basic Thrusters1 : scars_library/Actuators/Basic Thrusters  SystemSampleTime=-1  Latency=0  AutoFrameSizeCalculation=off
  Basic Thrusters2 : scars_library/Actuators/Basic Thrusters  SystemSampleTime=-1  Latency=0  AutoFrameSizeCalculation=off
  Constant : Constant  Value=thruster.distance
  Demux : Demux  Outputs=3
  Mux : Mux  Inputs=3
  Product : Product
  Sum : Sum  Inputs=+++
  Torque : Outport
  Power : Outport  Port=2
  wires:
  In1/1 -> Demux/1
  Demux/1 -> Basic Thrusters/1
  Basic Thrusters/1 -> Mux/1
  Basic Thrusters1/1 -> Mux/2
  Basic Thrusters2/1 -> Mux/3
  Basic Thrusters/2 -> Sum/1
  Basic Thrusters2/2 -> Sum/3
  Basic Thrusters1/2 -> Sum/2
  Constant/1 -> Product/2
  Mux/1 -> Product/1
  Product/1 -> Torque/1
  Sum/1 -> Power/1
  Demux/2 -> Basic Thrusters1/1
  Demux/3 -> Basic Thrusters2/1

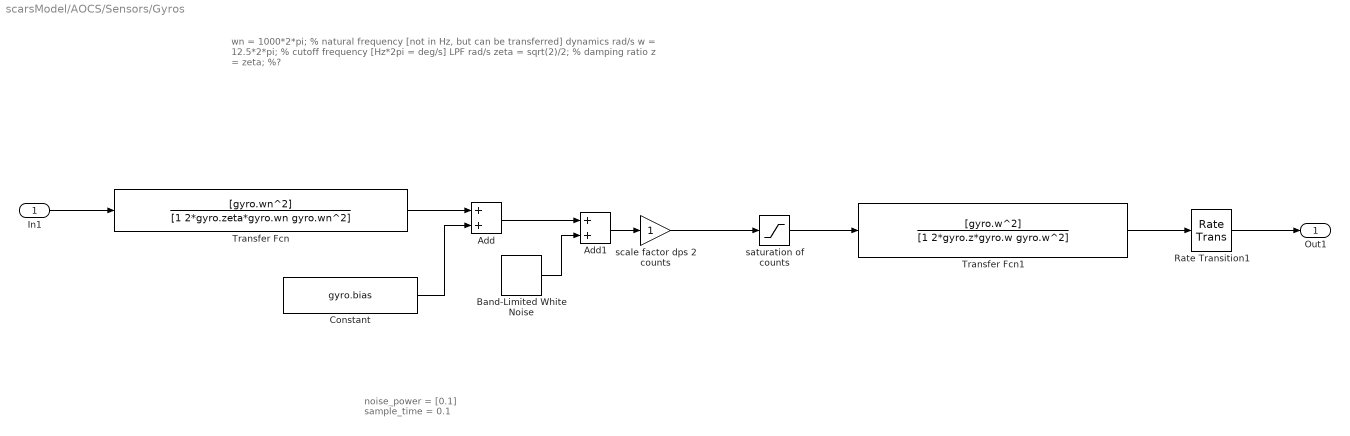
== system scarsModel/AOCS/Sensors/Gyros ==
  note: noise_power  = [0.1]
      | sample_time = 0.1
  note: wn = 1000*2*pi; % natural frequency [not in Hz, but can be transferred] dynamics rad/s
      | w = 12.5*2*pi; % cutoff frequency [Hz*2pi = deg/s] LPF rad/s
      | zeta = sqrt(2)/2; % damping ratio
      | z = zeta; %?
  In1 : Inport
  Add : Sum
  Add1 : Sum
  Band-Limited White Noise : simulink/Sources/Band-Limited White Noise  Cov=[gyro.noise_power]  Ts=gyro.sample_time  seed=[23341]
  Constant : Constant  Value=gyro.bias
  Rate Transition1 : RateTransition  OutPortSampleTime=gyro.rate
  Transfer Fcn : TransferFcn  Numerator=[gyro.wn^2]  Denominator=[1 2*gyro.zeta*gyro.wn gyro.wn^2]
  Transfer Fcn1 : TransferFcn  Numerator=[gyro.w^2]  Denominator=[1 2*gyro.z*gyro.w gyro.w^2]
  saturation of counts : Saturate  UpperLimit=gyro.max  LowerLimit=gyro.min
  scale factor dps 2 counts : Gain
  Out1 : Outport
  wires:
  Transfer Fcn/1 -> Add/1
  Constant/1 -> Add/2
  Add/1 -> Add1/1
  Band-Limited White Noise/1 -> Add1/2
  Add1/1 -> scale factor dps 2 counts/1
  scale factor dps 2 counts/1 -> saturation of counts/1
  saturation of counts/1 -> Transfer Fcn1/1
  Transfer Fcn1/1 -> Rate Transition1/1
  In1/1 -> Transfer Fcn/1
  Rate Transition1/1 -> Out1/1

== system scarsModel/Environment /Forces Environment/Subsystem ==
  Bus Element In : Inport  PortName=SatStates  Element=X_ECEF
  Spherical Harmonic Gravity Model1 : aerolibgravity2/Spherical Harmonic Gravity Model  units=Metric (MKS)  degree=120  action=Warning  ptype=EGM2008  datafile='aerogmm2b.mat'
      settings: SourceProductName=Aerospace Blockset  SourceProductBaseCode=AE
  To Workspace13 : ToWorkspace  VariableName=g  SampleTime=-1
  Out1 : Outport
  wires:
  Bus Element In/1 -> Spherical Harmonic Gravity Model1/1
  Spherical Harmonic Gravity Model1/1 -> Out1/1, To Workspace13/1
